simulink model "model_12_continuous"  (Simulink 8.7)
settings: Solver=VariableStepAuto  StartTime=0.0  StopTime=100  RelTol=1e-3
values from neighbouring files (symbols this model uses):
  den_f = dict_frac_f('denominator')    [simulate_model_continuous_debit.m]    (also in simulate_model_debit.m)
  den_r = dict_frac_r('denominator')    [simulate_model_continuous_debit.m]    (also in simulate_model_debit.m)
  num_f = dict_frac_f('nominator')    [simulate_model_continuous_debit.m]    (also in simulate_model_debit.m)
  num_r = dict_frac_r('nominator')    [simulate_model_continuous_debit.m]    (also in simulate_model_debit.m)
settings Model: Creator=danba  LastModifiedBy=danba
settings DataIOCC: LimitDataPoints=off  SaveFormat=Dataset
settings DebuggingCC: UnderspecifiedInitializationDetection=Simplified  MergeDetectMultiDrivingBlocksExec=error
settings HardwareCC: ProdBitPerPointer=64  ProdLargestAtomicFloat=Float  ProdIntDivRoundTo=Zero  ProdEndianess=LittleEndian  ProdWordSize=64  ProdHWDeviceType=Intel->x86-64 (Windows64)
settings ModelReferenceCC: PropagateSignalLabelsOutOfModel=on
settings ConfigComp: CovModelRefEnable=off

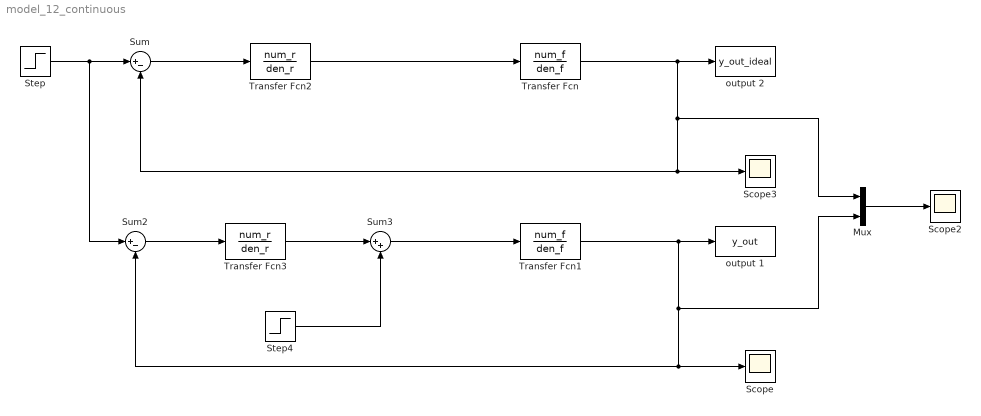
== system model_12_continuous ==
  Mux : Mux  Inputs=2
  Scope : Scope
  Scope2 : Scope
  Scope3 : Scope
  Step : Step  SampleTime=0.01
  Step4 : Step  Time=3  After=0.2  SampleTime=1
  Sum : Sum  Inputs=|+-
  Sum2 : Sum  Inputs=|+-
  Sum3 : Sum  Inputs=|++
  Transfer Fcn : TransferFcn  Numerator=num_f  Denominator=den_f
  Transfer Fcn1 : TransferFcn  Numerator=num_f  Denominator=den_f
  Transfer Fcn2 : TransferFcn  Numerator=num_r  Denominator=den_r
  Transfer Fcn3 : TransferFcn  Numerator=num_r  Denominator=den_r
  output 1 : ToWorkspace  VariableName=y_out  SaveFormat=Structure With Time  SampleTime=-1
  output 2 : ToWorkspace  VariableName=y_out_ideal  SaveFormat=Structure With Time  SampleTime=-1
  wires:
  Transfer Fcn2/1 -> Transfer Fcn/1
  Sum/1 -> Transfer Fcn2/1
  Sum2/1 -> Transfer Fcn3/1
  Transfer Fcn3/1 -> Sum3/1
  Sum3/1 -> Transfer Fcn1/1
  Step4/1 -> Sum3/2
  Mux/1 -> Scope2/1
  Transfer Fcn/1 -> output 2/1, Sum/2, Scope3/1, Mux/1
  Step/1 -> Sum2/1, Sum/1
  Transfer Fcn1/1 -> Sum2/2, Scope/1, Mux/2, output 1/1
